simulink model "AdaptiveCVSG"  (R2024b)
settings: Solver=ode4  StartTime=0.0  StopTime=60  FixedStep=1e-5  RelTol=1e-3
values from neighbouring files (symbols this model uses):
  mu = [6.21887134042 12.8843826697 23.6426615734 36.1444015647 49.5413580793 62.7022204476 75.4864006017 87.7683458466 99.0601107857 109.575241947 118.563685645 126.700169925 ... (200 elements, 1x200)]    [ann_model_params.mat]
  sigma = [10.4496327183 11.1148041158 11.7472409052 11.8906256492 12.3094874175 12.8461052911 13.270989651 13.5844531441 13.6128801345 13.7374243761 13.6590800387 13.618168837 ... (200 elements, 1x200)]    [ann_model_params.mat]
undefined symbols (not defined in the file or in its folder): Filter, Ls, params
libraries: neural x14, spsCurrentMeasurementLib x6, spsParallelRLCBranchLib x6, spsIGBTDiodeLib x6, spsSeriesRLCBranchLib x6, simulink x4, spsVoltageMeasurementLib x4, spsVariableInductorLib x3, spsVariableResistorLib x3, spsMeanLib x2, spsDCVoltageSourceLib x1, spsThreePhaseSourceLib x1
(part 4 of 4)

== system AdaptiveCVSG/ANN_based GIE/Feed-Forward Neural Network/Layer 2/Delays 1 ==
  "p{2}" : Inport  PortDimensions=8
      mask Display: e = 0.06;c1 = [120 230 180]/255;c2 = ([120 230 180]+0)/(256+128);c3 = ([120 230 180]+128)/(256+128);patch([0 1 1 0],[0 0 1 1],c1);patch([0 1 1 1-e 1-e 0+e],[0 0 1 1-e 0+e 0+e],c2);patch([0 0 1 1-e 0+e 0+e],[0 1 1 1-e 1-e 0+e],c3);plot([0 1 1 0 0],[0 0 1 1 0]);
  mux : Mux  Inputs=1
      mask Display: e = 0.06;c1 = [120 150 230]/255;c2 = ([120 150 230]+0)/383;c3 = ([120 150 230]+128)/383;patch([0 1 1 0],[0 0 1 1],c1);patch([0 1 1 1-e 1-e 0+e],[0 0 1 1-e 0+e 0+e],c2);patch([0 0 1 1-e 0+e 0+e],[0 1 1 1-e 1-e 0+e],c3);plot([0 1 1 0 0],[0 0 1 1 0]);disp('Mux')
  "pd{2,1}" : Outport
      mask Display: e = 0.06;c1 = [120 230 180]/255;c2 = ([120 230 180]+0)/(256+128);c3 = ([120 230 180]+128)/(256+128);patch([0 1 1 0],[0 0 1 1],c1);patch([0 1 1 1-e 1-e 0+e],[0 0 1 1-e 0+e 0+e],c2);patch([0 0 1 1-e 0+e 0+e],[0 1 1 1-e 1-e 0+e],c3);plot([0 1 1 0 0],[0 0 1 1 0]);
  wires:
  "p{2}"/1 -> mux/1
  mux/1 -> "pd{2,1}"/1

== system AdaptiveCVSG/ANN_based GIE/Feed-Forward Neural Network/Layer 2/LW{2,1} ==
  "ad{2,1}" : Inport  PortDimensions=8
      mask Display: e = 0.06;c1 = [120 230 180]/255;c2 = ([120 230 180]+0)/(256+128);c3 = ([120 230 180]+128)/(256+128);patch([0 1 1 0],[0 0 1 1],c1);patch([0 1 1 1-e 1-e 0+e],[0 0 1 1-e 0+e 0+e],c2);patch([0 0 1 1-e 0+e 0+e],[0 1 1 1-e 1-e 0+e],c3);plot([0 1 1 0 0],[0 0 1 1 0]);
  "IW{2,1}(1,:)'" : Constant  Value=[0.1312871511283932590696821307574282400310039520263671875;-0.5972369254694636087066328400396741926670074462890625;0.272093265660533878413929187445319257676601409912109375;0.28991588457986428029045100629446096718311309814453125;0.1284042379428932123541784449116676114499568939208984375;0.55391103847346123689732166894827969372272491455078125;0.719319174309459352656404007575474679470062255859375;0.140185906659878067870295126340351998805999755859375]
      mask Display: e = 0.06;c1 = [120 150 230]/255;c2 = ([120 150 230]+0)/383;c3 = ([120 150 230]+128)/383;patch([0 1 1 0],[0 0 1 1],c1);patch([0 1 1 1-e 1-e 0+e],[0 0 1 1-e 0+e 0+e],c2);patch([0 0 1 1-e 0+e 0+e],[0 1 1 1-e 1-e 0+e],c3);plot([0 1 1 0 0],[0 0 1 1 0]);disp('weights');
  "IW{2,1}(2,:)'" : Constant  Value=[0.1445753503799891703796021147354622371494770050048828125;-0.5923321763649835869358639683923684060573577880859375;0.271417858112287413430152582805021665990352630615234375;0.2816351479369736399149815042619593441486358642578125;0.11179711101264923345244284291766234673559665679931640625;0.563227466159649026167244301177561283111572265625;0.7093268586162413402718129873392172157764434814453125;0.138216632818150941819368426877190358936786651611328125]
      mask Display: e = 0.06;c1 = [120 150 230]/255;c2 = ([120 150 230]+0)/383;c3 = ([120 150 230]+128)/383;patch([0 1 1 0],[0 0 1 1],c1);patch([0 1 1 1-e 1-e 0+e],[0 0 1 1-e 0+e 0+e],c2);patch([0 0 1 1-e 0+e 0+e],[0 1 1 1-e 1-e 0+e],c3);plot([0 1 1 0 0],[0 0 1 1 0]);disp('weights');
  Mux : Mux  Inputs=2
      mask Display: e = 0.06;c1 = [120 150 230]/255;c2 = ([120 150 230]+0)/383;c3 = ([120 150 230]+128)/383;patch([0 1 1 0],[0 0 1 1],c1);patch([0 1 1 1-e 1-e 0+e],[0 0 1 1-e 0+e 0+e],c2);patch([0 0 1 1-e 0+e 0+e],[0 1 1 1-e 1-e 0+e],c3);plot([0 1 1 0 0],[0 0 1 1 0]);disp('Mux');
  dotprod1 : neural/Weight Functions/dotprod
  dotprod2 : neural/Weight Functions/dotprod
  "lz{2,1}" : Outport
      mask Display: e = 0.06;c1 = [120 230 180]/255;c2 = ([120 230 180]+0)/(256+128);c3 = ([120 230 180]+128)/(256+128);patch([0 1 1 0],[0 0 1 1],c1);patch([0 1 1 1-e 1-e 0+e],[0 0 1 1-e 0+e 0+e],c2);patch([0 0 1 1-e 0+e 0+e],[0 1 1 1-e 1-e 0+e],c3);plot([0 1 1 0 0],[0 0 1 1 0]);
  wires:
  "IW{2,1}(1,:)'"/1 -> dotprod1/1
  "ad{2,1}"/1 -> dotprod1/2, dotprod2/2
  dotprod1/1 -> Mux/1
  "IW{2,1}(2,:)'"/1 -> dotprod2/1
  dotprod2/1 -> Mux/2
  Mux/1 -> "lz{2,1}"/1

== matlab function AdaptiveCVSG/Grid impedance1/Train2 ==
  data: t input; Lg output
function Lg = fcn(t)
    %— Tham số hệ thống ———————————————————————————————————
    Vll_rms = 110*sqrt(3);
    P_rated = 5000;
    w0       = 2*pi*50;

    %— Hồ sơ SCR & thời gian bước —————————————————————————
    persistent scr_vec step_T n_step
    if isempty(scr_vec)
        scr_vec = [2, 8, 20];
        step_T  = 20.0;            % mỗi bước 20 s
        n_step  = numel(scr_vec);
    end

    %— Chọn chỉ số bước bằng ceil ——————————————————————
    if t <= 0
        idx = 1;
    else
        idx = ceil(t / step_T);
        if idx > n_step
            idx = n_step;
        end
    end
    scr = scr_vec(idx);

    %— Tính Lg từ SCR —————————————————————————————
    Lg = Vll_rms^2 / ( scr * P_rated * w0 );
end

== matlab function AdaptiveCVSG/Grid impedance1/Train1 ==
  data: Lg input; Rg output
function Rg = fcn(Lg)
f0 = 50;
XR = 1;
Rg = 2*pi*f0*Lg/XR;
